simulink model "ssc1"  (R2017b)
settings: Solver=VariableStepAuto  StartTime=0.0  StopTime=5  MaxStep=1e-4  RelTol=1e-3
undefined symbols (not defined in the file): Ion, Lithium
libraries: powerlib x30, simulink x10, electricdrivelib x4
settings Model: SnapshotBufferSize=100000000  SnapshotInterval=100000000  Creator=OCAK5596  LastModifiedBy=Ocak5596

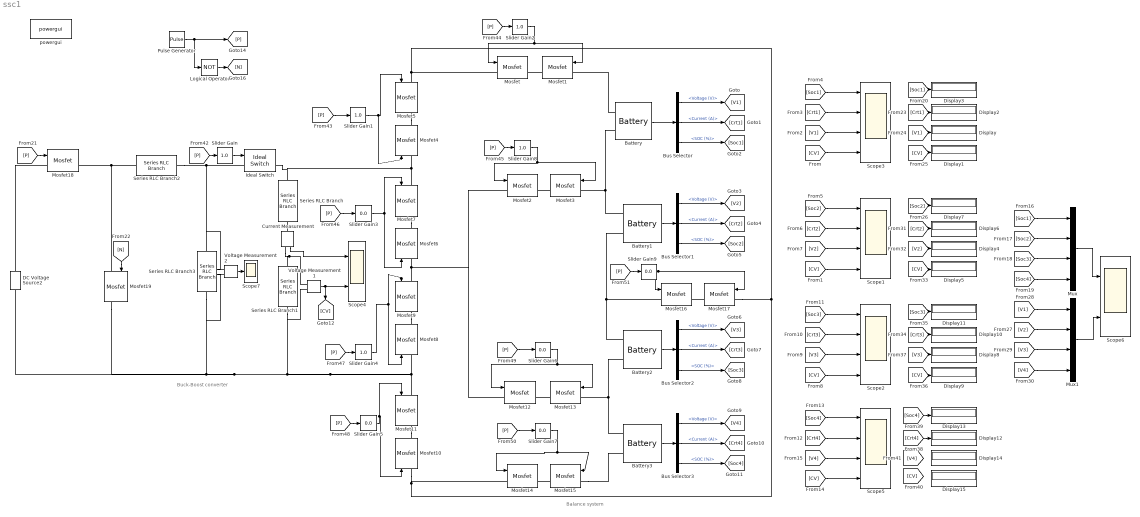
== system ssc1 ==
  note: Balance system
  note: Buck-Boost converter
  Battery : electricdrivelib/Extra Sources/Battery  BatType=Lithium-Ion  ShowTempParam=off  ThermalPreset=no  ShowAgeParam=off  NomV=3.3  NomQ=2.3  SOC=20  Batt_Tr=1e-3  PresetModel=on  MaxQ=2.3  MinV=2.475  FullV=3.8412  Dis_rate=1  R=0.014348  Normal_OP=2.08  expZone="[3.5653       0.113]"  current=[6.5 13 32.5]  Units=Time  Tci=20  NomT=20  T2=-30  MaxQ2=4.8  FullV2=7.1  Normal_OP2=5.655  expZone2="[6.58           1]"  Rca=0.6  ti=2000  Dp=0  Neq0=0  Tsim=1e6  Ta1=25  Qeol=5.4*0.9  Reol=0.013333*1.2  Char_age=[2.3478, 3]  Dis_age=[2.3478, 10]  N1=1500  N2=10500  N3=1000  N4=1400  Ta2=45  N5=950
  Battery1 : electricdrivelib/Extra Sources/Battery  BatType=Lithium-Ion  ShowTempParam=off  ThermalPreset=no  ShowAgeParam=off  NomV=3.3  NomQ=20  SOC=80  Batt_Tr=30  PresetModel=on  MaxQ=20  MinV=2.475  FullV=3.8412  Dis_rate=8.6957  R=0.00165  Normal_OP=18.087  expZone="[3.5653     0.98261]"  current=[6.5 13 32.5]  Units=Time  Tci=20  NomT=20  T2=-30  MaxQ2=4.8  FullV2=7.1  Normal_OP2=5.655  expZone2="[6.58           1]"  Rca=0.6  ti=2000  Dp=0  Neq0=0  Tsim=1e6  Ta1=25  Qeol=5.4*0.9  Reol=0.013333*1.2  Char_age=[2.3478, 3]  Dis_age=[2.3478, 10]  N1=1500  N2=10500  N3=1000  N4=1400  Ta2=45  N5=950
  Battery2 : electricdrivelib/Extra Sources/Battery  BatType=Lithium-Ion  ShowTempParam=off  ThermalPreset=no  ShowAgeParam=off  NomV=3.3  NomQ=2.3  SOC=20  Batt_Tr=1e-5  PresetModel=on  MaxQ=2.3  MinV=2.475  FullV=3.8412  Dis_rate=1  R=0.014348  Normal_OP=2.08  expZone="[3.5653       0.113]"  current=[6.5 13 32.5]  Units=Time  Tci=20  NomT=20  T2=-30  MaxQ2=4.8  FullV2=7.1  Normal_OP2=5.655  expZone2="[6.58           1]"  Rca=0.6  ti=2000  Dp=0  Neq0=0  Tsim=1e6  Ta1=25  Qeol=5.4*0.9  Reol=0.013333*1.2  Char_age=[2.3478, 3]  Dis_age=[2.3478, 10]  N1=1500  N2=10500  N3=1000  N4=1400  Ta2=45  N5=950
  Battery3 : electricdrivelib/Extra Sources/Battery  BatType=Lithium-Ion  ShowTempParam=off  ThermalPreset=no  ShowAgeParam=off  NomV=3.3  NomQ=2.3  SOC=20  Batt_Tr=1e-5  PresetModel=on  MaxQ=2.3  MinV=2.475  FullV=3.8412  Dis_rate=1  R=0.014348  Normal_OP=2.08  expZone="[3.5653       0.113]"  current=[6.5 13 32.5]  Units=Time  Tci=20  NomT=20  T2=-30  MaxQ2=4.8  FullV2=7.1  Normal_OP2=5.655  expZone2="[6.58           1]"  Rca=0.6  ti=2000  Dp=0  Neq0=0  Tsim=1e6  Ta1=25  Qeol=5.4*0.9  Reol=0.013333*1.2  Char_age=[2.3478, 3]  Dis_age=[2.3478, 10]  N1=1500  N2=10500  N3=1000  N4=1400  Ta2=45  N5=950
  Bus Selector{,1..3} (4 alike) : BusSelector  OutputSignals=Voltage (V),Current (A),SOC (%)
  Current Measurement : powerlib/Measurements/Current Measurement  PhasorSimulation=off  OutputType=Complex  PSBequivalent=0
  DC Voltage Source2 : powerlib/Electrical Sources/DC Voltage Source  Amplitude=15  Measurements=Voltage
  Display{,1..15} (16 alike) : Display
  Ideal Switch : powerlib/Power Electronics/Ideal Switch  Ron=0.001  Lon=0  IC=0  Rs=1e5  Cs=inf  Measurements=on
  Logical Operator : Logic  Operator=NOT  AllPortsSameDT=off  OutDataTypeStr=boolean
  Mosfet{,1..17} (18 alike) : powerlib/Power Electronics/Mosfet  Ron=0.0048  Lon=0  Rd=0.01  Vfd=0  IC=0  Rs=1e5  Cs=inf  Measurements=on
  Mosfet18 : powerlib/Power Electronics/Mosfet  Ron=0.1  Lon=0  Rd=0.01  Vfd=0  IC=0  Rs=1e5  Cs=inf  Measurements=on
  Mosfet19 : powerlib/Power Electronics/Mosfet  Ron=0.1  Lon=0  Rd=0.01  Vfd=0  IC=0  Rs=1e5  Cs=inf  Measurements=on
  Mux : Mux
  Mux1 : Mux
  Pulse Generator : DiscretePulseGenerator  PulseType=Time based  Period=1/500  PulseWidth=90
  Scope{1..3,5} (4 alike) : Scope  NumInputPorts=4
  Scope4 : Scope  NumInputPorts=2
  Scope6 : Scope  NumInputPorts=2
  Scope7 : Scope
  Series RLC Branch : powerlib/Elements/Series RLC Branch  LConnTagsString=__new0  RConnTagsString=__new0  BranchType=R  Resistance=1  Inductance=1e-3  SetiL0=off  InitialCurrent=0  Capacitance=1e-6  Setx0=off  InitialVoltage=0  Measurements=None
  Series RLC Branch1 : powerlib/Elements/Series RLC Branch  LConnTagsString=__new0  RConnTagsString=__new0  BranchType=C  Resistance=1  Inductance=1e-3  SetiL0=off  InitialCurrent=0  Capacitance=0.022  Setx0=off  InitialVoltage=15  Measurements=Branch voltage and current
  Series RLC Branch2 : powerlib/Elements/Series RLC Branch  LConnTagsString=__new0  RConnTagsString=__new0  BranchType=RL  Resistance=0.1  Inductance=1e-3  SetiL0=off  InitialCurrent=0  Capacitance=1e-6  Setx0=off  InitialVoltage=0  Measurements=None
  Series RLC Branch3 : powerlib/Elements/Series RLC Branch  LConnTagsString=__new0  RConnTagsString=__new0  BranchType=RC  Resistance=0.001  Inductance=1e-3  SetiL0=off  InitialCurrent=0  Capacitance=1000e-6  Setx0=off  InitialVoltage=0  Measurements=None
  Slider Gain{,1..2,4,8} (5 alike) : simulink/Math Operations/Slider Gain  gain=1.0  low=0  high=1
  Slider Gain{3,5..7,9} (5 alike) : simulink/Math Operations/Slider Gain  gain=0.0  low=0  high=1
  Voltage Measurement1 : powerlib/Measurements/Voltage Measurement  PhasorSimulation=off  OutputType=Complex  PSBequivalent=0
  Voltage Measurement2 : powerlib/Measurements/Voltage Measurement  PhasorSimulation=off  OutputType=Complex  PSBequivalent=0
  powergui : powerlib/powergui  Priority=1  SimulationMode=Continuous  SampleTime=1e-3  frequency=60  Iterations=50  frequencyindice=0  Pbase=100e6  ErrMax=1e-4  UnitsV=kV  UnitsW=MW  buscounter=0  FunctionMessages=off  echomessages=off  EnableUseOfTLC=off  CurrentSourceSwitches=off  DisableSnubberDevices=off  DisableRonSwitches=off  DisableVfSwitches=off  DisplayEquations=off  SolverType=Tustin/Backward Euler (TBE)  Interpol=off  ExternalGateDelay=off  methode=off  Ts=100  x0status=blocks  SPID=on  SwTol=0  HookPort=off  RestoreLinks=warning  ResistiveCurrentMeasurement=off  Frange=[0:2:500]  Ylog=off  Xlog=on  ShowGrid=off  save=off  variable=ZData  structure=0  ZoomFFT=off  StartTime=0.0  cycles=1  DisplayStyle=1  fundamental=60  FreqAxis=off  MaxFrequency=1000  frequencyindicesteady=1  RmsSteady=1  display=off
  wires:
  Battery/1 -> Bus Selector/1
  Battery1/1 -> Bus Selector1/1
  Bus Selector/1 -> [V1]  "<Voltage (V)>"
  Bus Selector/2 -> [Crt1]  "<Current (A)>"
  Bus Selector/3 -> [Soc1]  "<SOC (%)>"
  Bus Selector1/1 -> [V2]  "<Voltage (V)>"
  Bus Selector1/2 -> [Crt2]  "<Current (A)>"
  Bus Selector1/3 -> [Soc2]  "<SOC (%)>"
  Bus Selector2/2 -> [Crt3]  "<Current (A)>"
  Bus Selector2/1 -> [V3]  "<Voltage (V)>"
  Battery2/1 -> Bus Selector2/1
  Bus Selector2/3 -> [Soc3]  "<SOC (%)>"
  Bus Selector3/2 -> [Crt4]  "<Current (A)>"
  Bus Selector3/1 -> [V4]  "<Voltage (V)>"
  Battery3/1 -> Bus Selector3/1
  Bus Selector3/3 -> [Soc4]  "<SOC (%)>"
  Voltage Measurement1/1 -> Scope4/2, [CV]
  [Soc1] -> Scope3/1
  [Crt1] -> Scope3/2
  Slider Gain4/1 -> Mosfet8/1, Mosfet9/1
  Current Measurement/1 -> Scope4/1
  [V1] -> Scope3/3
  [CV] -> Scope3/4
  [CV] -> Scope1/4
  [V2] -> Scope1/3
  [Crt2] -> Scope1/2
  [Soc2] -> Scope1/1
  [Soc3] -> Scope2/1
  [Crt3] -> Scope2/2
  [V3] -> Scope2/3
  [CV] -> Scope2/4
  [CV] -> Scope5/4
  [V4] -> Scope5/3
  [Crt4] -> Scope5/2
  [Soc4] -> Scope5/1
  [Soc1] -> Mux/1
  [Soc2] -> Mux/2
  [Soc3] -> Mux/3
  [Soc4] -> Mux/4
  Mux/1 -> Scope6/1
  Pulse Generator/1 -> [P], Logical Operator/1
  Logical Operator/1 -> [N]
  Mux1/1 -> Scope6/2
  [V2] -> Mux1/2
  [V1] -> Mux1/1
  [V3] -> Mux1/3
  [V4] -> Mux1/4
  [P] -> Mosfet18/1
  [N] -> Mosfet19/1
  Voltage Measurement2/1 -> Scope7/1
  Slider Gain3/1 -> Mosfet6/1, Mosfet7/1
  Slider Gain6/1 -> Mosfet13/1, Mosfet12/1
  Slider Gain7/1 -> Mosfet14/1, Mosfet15/1
  Slider Gain5/1 -> Mosfet10/1, Mosfet11/1
  [V1] -> Display/1
  [CV] -> Display1/1
  [V3] -> Display8/1
  [Crt3] -> Display10/1
  [Soc3] -> Display11/1
  [CV] -> Display9/1
  [CV] -> Display5/1
  [V2] -> Display4/1
  [Crt2] -> Display6/1
  [Soc2] -> Display7/1
  [Soc1] -> Display3/1
  [Crt1] -> Display2/1
  [Soc4] -> Display13/1
  [Crt4] -> Display12/1
  [P] -> Slider Gain/1
  Slider Gain/1 -> Ideal Switch/1
  [P] -> Slider Gain1/1
  [P] -> Slider Gain2/1
  Slider Gain1/1 -> Mosfet4/1, Mosfet5/1
  [P] -> Slider Gain3/1
  [P] -> Slider Gain4/1
  [P] -> Slider Gain5/1
  [P] -> Slider Gain6/1
  [P] -> Slider Gain7/1
  [P] -> Slider Gain8/1
  Slider Gain8/1 -> Mosfet3/1, Mosfet2/1
  [P] -> Slider Gain9/1
  Slider Gain9/1 -> Mosfet17/1, Mosfet16/1
  Slider Gain2/1 -> Mosfet/1, Mosfet1/1
  connections:
  Mosfet1/RConn1 -- Mosfet/RConn1
  Mosfet3/RConn1 -- Mosfet2/RConn1
  Mosfet5/RConn1 -- Mosfet4/RConn1
  Mosfet7/RConn1 -- Mosfet6/RConn1
  Mosfet7/LConn1 -- Ideal Switch/RConn1 -- Series RLC Branch/LConn1 -- Mosfet4/LConn1
  Mosfet11/RConn1 -- Mosfet10/RConn1
  Mosfet9/RConn1 -- Mosfet8/RConn1
  Mosfet9/LConn1 -- Mosfet2/LConn1 -- Mosfet12/LConn1 -- Mosfet6/LConn1
  Mosfet10/LConn1 -- Mosfet14/LConn1 -- Mosfet17/LConn1 -- Mosfet/LConn1 -- Mosfet5/LConn1
  Mosfet13/RConn1 -- Mosfet12/RConn1
  Mosfet15/RConn1 -- Mosfet14/RConn1
  Battery/LConn1 -- Mosfet1/LConn1
  Battery/LConn2 -- Mosfet3/LConn1 -- Battery1/LConn1
  Mosfet17/RConn1 -- Mosfet16/RConn1
  Mosfet16/LConn1 -- Battery2/LConn1 -- Battery1/LConn2
  Battery2/LConn2 -- Battery3/LConn1 -- Mosfet13/LConn1
  Mosfet15/LConn1 -- Battery3/LConn2
  Voltage Measurement1/LConn1 -- Current Measurement/RConn1 -- Series RLC Branch1/LConn1
  Series RLC Branch/RConn1 -- Current Measurement/LConn1
  Mosfet18/LConn1 -- DC Voltage Source2/RConn1
  Mosfet19/LConn1 -- Mosfet18/RConn1 -- Series RLC Branch2/LConn1
  Mosfet11/LConn1 -- Voltage Measurement1/LConn2 -- Series RLC Branch1/RConn1 -- Voltage Measurement2/LConn2 -- Series RLC Branch3/RConn1 -- Mosfet19/RConn1 -- DC Voltage Source2/LConn1 -- Mosfet8/LConn1
  Series RLC Branch2/RConn1 -- Voltage Measurement2/LConn1 -- Series RLC Branch3/LConn1 -- Ideal Switch/LConn1
